simulink model "Toggel"  (R2024b)
settings: Solver=VariableStepAuto  StartTime=0.0  StopTime=inf  MaxStep=1e-3  RelTol=1e-3
undefined symbols (not defined in the file): a1, a2, a3, initial, k_w, Kd, Ki, Kp, lower_sat, tau_w, upper_sat
libraries: simulink x1, slpidlib x1
settings Model: Creator=elias  LastModifiedBy=elias

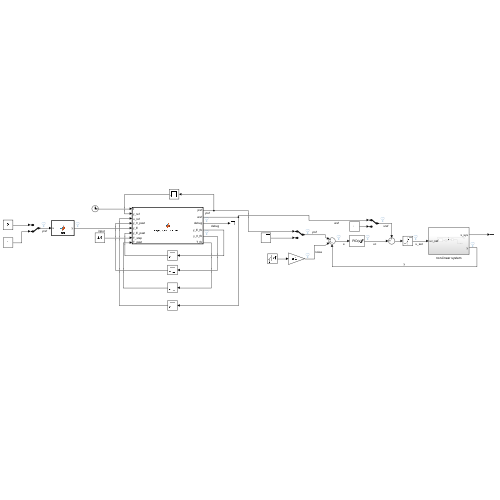
[thumbnail: Simulink's stored preview of the top-level diagram]
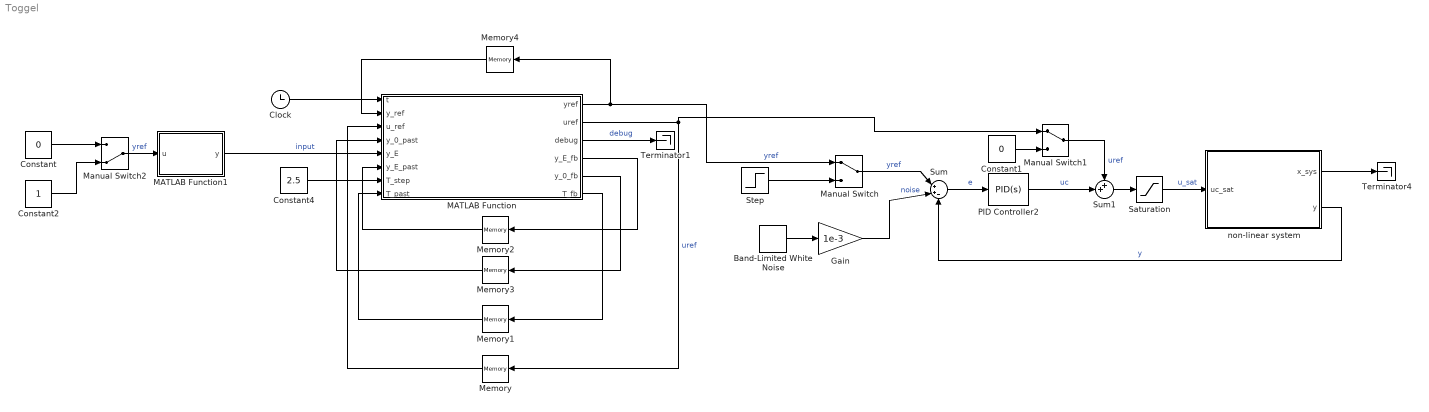
== system Toggel ==
  Band-Limited White Noise : simulink/Sources/Band-Limited White Noise  Cov=[0.1]  Ts=0.1  seed=[23341]
  Clock : Clock
  Constant : Constant  Value=0
  Constant1 : Constant  Value=0
  Constant2 : Constant
  Constant4 : Constant  Value=2.5
  Gain : Gain  Gain=1e-3
  MATLAB Function : MATLAB Function  TreatAsAtomicUnit=on
  MATLAB Function1 : MATLAB Function  TreatAsAtomicUnit=on
  Manual Switch : ManualSwitch
  Manual Switch1 : ManualSwitch
  Manual Switch2 : ManualSwitch  CurrentSetting=0
  Memory : Memory
  Memory1 : Memory
  Memory2 : Memory
  Memory3 : Memory  InitialCondition=initial(1)
  Memory4 : Memory  InitialCondition=initial(1)
  PID Controller2 : slpidlib/PID Controller  Controller=PID  Form=Parallel  TimeDomain=Continuous-time  UseExternalTs=off  SampleTime=-1  IntegratorMethod=Forward Euler  FilterMethod=Forward Euler  ControllerParametersSource=internal  P=Kp  I=Ki  UseKiTs=off  D=Kd  UseExternalDerivativeSource=off  N=100  UseFilter=on  TunerSelectOption=Transfer Function Based (PID Tuner App)  InitialConditionSource=internal  InitialConditionForIntegrator=0  InitialConditionForFilter=0  DifferentiatorICPrevScaledInput=0  ExternalReset=none  TrackingMode=off  Kt=1  LimitOutput=on  SatLimitsSource=internal  UpperSaturationLimit=inf  LowerSaturationLimit=-inf  LinearizeAsGain=on  AntiWindupMode=clamping  Kb=1  LimitIntegrator=off  UpperIntegratorSaturationLimit=inf  LowerIntegratorSaturationLimit=-inf  POutMin=[]  POutMax=[]  IOutMin=[]  IOutMax=[]  DOutMin=[]  DOutMax=[]  NOutMin=[]  NOutMax=[]  SumOutMin=[]  SumOutMax=[]  SaturationOutMin=[]  SaturationOutMax=[]  PParamMin=[]  PParamMax=[]  IParamMin=[]  IParamMax=[]  DParamMin=[]  DParamMax=[]  NParamMin=[]  NParamMax=[]  KbParamMin=[]  KbParamMax=[]  KtParamMin=[]  KtParamMax=[]  KbOutMin=[]  KbOutMax=[]  KtOutMin=[]  KtOutMax=[]  IntegratorOutMin=[]  IntegratorOutMax=[]  FilterOutMin=[]  FilterOutMax=[]  SumI1OutMin=[]  SumI1OutMax=[]  SumI2OutMin=[]  SumI2OutMax=[]  SumI3OutMin=[]  SumI3OutMax=[]  SumI4OutMin=[]  SumI4OutMax=[]  SumDOutMin=[]  SumDOutMax=[]  DifferentiatorOutMin=[]  DifferentiatorOutMax=[]  FilterDiffOutCoefMin=[]  FilterDiffOutCoefMax=[]  ReciprocalOutMin=[]  ReciprocalOutMax=[]  SumDenOutMin=[]  SumDenOutMax=[]  SumNumOutMin=[]  SumNumOutMax=[]  DivideOutMin=[]  DivideOutMax=[]  UdiffTsProdOutMin=[]  UdiffTsProdOutMax=[]  NTsProdOutMin=[]  NTsProdOutMax=[]  UintegralTsProdOutMin=[]  UintegralTsProdOutMax=[]  UngainTsProdOutMin=[]  UngainTsProdOutMax=[]  ClampingZeroOutDataTypeStr=Inherit: Inherit via back propagation  ClampingZeroOutMin=[]  ClampingZeroOutMax=[]  FilterDenConstantOutDataTypeStr=Inherit: Inherit via back propagation  FilterDenConstantOutMin=[]  FilterDenConstantOutMax=[]  PCopyOutDataTypeStr=Inherit: Inherit via back propagation  PCopyOutMin=[]  PCopyOutMax=[]  NCopyOutDataTypeStr=Inherit: Inherit via back propagation  NCopyOutMin=[]  NCopyOutMax=[]  IntegratorContinuousStateAttributes=''  IntegratorStateMustResolveToSignalObject=off  IntegratorRTWStateStorageClass=Auto  FilterContinuousStateAttributes=''  FilterStateMustResolveToSignalObject=off  FilterRTWStateStorageClass=Auto  ParallelPVariant=InternalParameters  IdealPVariant=Disabled  IVariant=InternalParameters  DVariant=InternalParameters  IntegratorVariant=Continuous  SatVariant=Enabled  AWVariant=ContClampingParallel  PCopyVariant=Disabled  TRVariant=Disabled  FdbkBlocksVariant=Forward  IdealPFdbkVariant=Disabled  SatFdbkVariant=Disabled  DerivativeFilterVariant=ContFilter  NVariant=InternalParameters  NCopyVariant=Disabled  FilterICVariant=InternalICsFilter  IntegratorICVariant=InternalICs  ExternalResetVariant=Disabled  TRSumVariant=Passthrough  SumFdbkVariant=Disabled  SumVariant=Sum_PID  TsampFilterVariant=InternalTs  TsampNgainVariant=Passthrough  TsampIntegralVariant=Disabled_SignalSpec  ExternalSaturationOutDataTypeStr=Inherit: Same as second input  DerivativeSourceVariant=ErrorSignal  PreIntVariant=InternalPreInt
  Saturation : Saturate  UpperLimit=5  LowerLimit=0
  Step : Step  SampleTime=0
  Sum : Sum  Inputs=|++-
  Sum1 : Sum  Inputs=++|
  Terminator1 : Terminator
  Terminator4 : Terminator
  non-linear system : Subsystem
  wires:
  Constant4/1 -> MATLAB Function/7(T_step)
  MATLAB Function1/1(y) -> MATLAB Function/5(y_E)  "input"
  PID Controller2/1 -> Sum1/2  "uc"
  Manual Switch/1 -> Sum/1  "yref"
  Gain/1 -> Sum/2  "noise"
  non-linear system/2(y) -> Sum/3  "y"
  Constant1/1 -> Manual Switch1/2
  Sum/1 -> PID Controller2/1  "e"
  Manual Switch1/1 -> Sum1/1  "uref"
  non-linear system/1(x_sys) -> Terminator4/1
  Step/1 -> Manual Switch/2
  Band-Limited White Noise/1 -> Gain/1
  Saturation/1 -> non-linear system/1(uc_sat)  "u_sat"
  Sum1/1 -> Saturation/1
  MATLAB Function/1(yref) -> Memory4/1, Manual Switch/1  "yref"
  MATLAB Function/2(uref) -> Memory/1, Manual Switch1/1  "uref"
  Clock/1 -> MATLAB Function/1(t)
  MATLAB Function/3(debug) -> Terminator1/1  "debug"
  MATLAB Function/4(y_E_fb) -> Memory2/1
  Memory2/1 -> MATLAB Function/6(y_E_past)
  MATLAB Function/5(y_0_fb) -> Memory3/1
  Memory3/1 -> MATLAB Function/4(y_0_past)
  Memory1/1 -> MATLAB Function/8(T_past)
  MATLAB Function/6(T_fb) -> Memory1/1
  Memory/1 -> MATLAB Function/3(u_ref)
  Memory4/1 -> MATLAB Function/2(y_ref)
  Manual Switch2/1 -> MATLAB Function1/1(u)  "yref"
  Constant/1 -> Manual Switch2/1
  Constant2/1 -> Manual Switch2/2

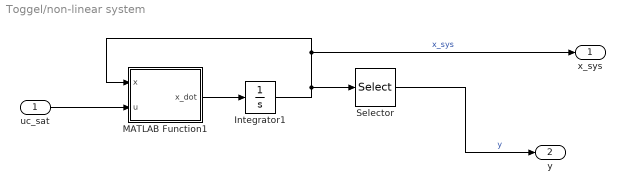
== system Toggel/non-linear system ==
  uc_sat : Inport
  Integrator1 : Integrator  InitialCondition=initial  LimitOutput=on  UpperSaturationLimit=upper_sat  LowerSaturationLimit=lower_sat
  MATLAB Function1 : MATLAB Function  TreatAsAtomicUnit=on
  Selector : Selector  InputPortWidth=3  IndexOptions=Index vector (dialog)  Indices=1  OutputSizes=1
  x_sys : Outport
  y : Outport  Port=2
  wires:
  Integrator1/1 -> Selector/1, MATLAB Function1/1(x), x_sys/1  "x_sys"
  MATLAB Function1/1(x_dot) -> Integrator1/1
  uc_sat/1 -> MATLAB Function1/2(u)
  Selector/1 -> y/1  "y"

== matlab function Toggel/non-linear system/MATLAB Function1 ==
  data: x input; u input; x_dot output; a1 parameter; a2 parameter; a3 parameter; tau_w parameter; k_w parameter
function x_dot  = fcn(x,u,a1, a2, a3, tau_w, k_w)



%nonlinear set of equation
x_dot = [x(2); (a1*x(3)-a2*x(2))^2-a3; -x(3)/tau_w]+[0; 0; k_w/tau_w]*u;

== matlab function Toggel/MATLAB Function ==
  data: yref output; uref output; t input; y_ref input; u_ref input; y_0_past input; y_E input; y_E_past input; T_step input; T_past input; tau_w parameter; a3 parameter; a2 parameter; a1 parameter; k_w parameter; debug output; y_E_fb output; y_0_fb output; T_fb output
function [yref, uref, debug, y_E_fb, y_0_fb, T_fb] = trajectory_planning(t, y_ref, u_ref, y_0_past, y_E, y_E_past, T_step, T_past, tau_w, a3, a2, a1, k_w)
    % t: Current simulation time
    % y_0: Initial height of the ball
    % y_T: Desired height of the ball
    % T: Duration of the trajectory
    % tau_w: Fan time constant
    % a3, a2, a1: System coefficients
    % k_w: Fan gain

   

    % Order of the system
    n = 3;

    if(y_E == y_E_past) % still in the same transition
        y_0 = y_0_past;
    else    % start of new transition
        y_0 = y_ref;
        T_past = t;
    end
    
     % Normalize the current time
    tau = (t-T_past) / T_step;
    
    if(t < T_past + T_step)
        % Initialize coefficient matrix
        phi = zeros(n+1, 2*n+2);
    
        % Fill the first row of the coefficient matrix
        for k = 0:n
        phi(1,n+1-k) = nchoosek(n,k)*(-1)^k/(n+k+1);
        end
        
        % Add factor (which is multiplied by the sum) to all coefficients
        phi = factorial(2*n+1)/factorial(n)^2*phi;
        
        for j = 1:n
        phi(j+1,j+1:end) = 1/T_step*polyder(phi(j,j:end));
        end
        
        phi4 = zeros(n+1,length(tau));
        
        for i = 1:n+1
            phi4(i,:) = polyval(phi(i,:),tau);
        end
        
        % Compute the scaled trajectory
        yf = (y_E - y_0) * phi4;
        yf(1) = y_0 + yf(1); % Add the initial height for the non-derived function
    
        % Compute the angular velocity and its derivative
        omega = (sqrt(yf(3) + a3) + a2 * yf(2)) / a1;
        omega_dot = (1/2) * 1 / sqrt(yf(3) + a3) * yf(4) / a1 + a2 / a1 * yf(3);
    
        % Compute the reference control input
        uref = (tau_w * omega_dot + omega) / k_w;
    
        % Output the current reference trajectory and control input
        yref = yf(1);
        debug = phi4(1);
    else
        uref = u_ref;
        yref = y_ref;
        debug = 0;
    end
    T_fb = T_past;
    y_0_fb = y_0;
    y_E_fb = y_E;
    
end

== matlab function Toggel/MATLAB Function1 ==
  data: u input; y output
function y = fcn(u)

if(u)
    y = 0.15;
else
    y = 0.2;
end
